simulink model "Simulatie"  (R2018b)
settings: Solver=FixedStepAuto  StartTime=0.0  StopTime=10  FixedStep=1e-5  RelTol=1e-3
values from neighbouring files (symbols this model uses):
  A = [-(bm*(n^2) + bg)/(Jm*(n^2) + Jg) Kt*n/(Jm*(n^2) + Jg) ... (first row only)    [DC_motor_geared_integral_discrete_sysid23.m]    (also in DC_motor_geared_lqr_discrete_sysid23.m; finalScript.m; finalScriptV2.m; precompensatorVSintegrator.m)
  Ad = sysdi.A    [DC_motor_geared_integral_discrete_sysid23.m]    (also in DC_motor_geared_lqr_discrete_sysid23.m = sysd.A; finalScript.m; finalScriptV2.m)
  B = [0 ... (first row only)    [DC_motor_geared_integral_discrete_sysid23.m]    (also in DC_motor_geared_lqr_discrete_sysid23.m; finalScript.m; finalScriptV2.m; precompensatorVSintegrator.m)
  Bd = sysdi.B    [DC_motor_geared_integral_discrete_sysid23.m]    (also in DC_motor_geared_lqr_discrete_sysid23.m = sysd.B; finalScript.m; finalScriptV2.m)
  C = [1 0]    [DC_motor_geared_integral_discrete_sysid23.m]    (also in DC_motor_geared_lqr_discrete_sysid23.m = eye(2); finalScript.m; finalScriptV2.m; precompensatorVSintegrator.m = eye(2))
  D = [0]    [DC_motor_geared_integral_discrete_sysid23.m]    (also in DC_motor_geared_lqr_discrete_sysid23.m = [0;0]; finalScript.m; finalScriptV2.m; precompensatorVSintegrator.m)
  Kc = lqr(sysd,Q,R)    [DC_motor_geared_lqr_discrete_sysid23.m]    (also in precompensatorVSintegrator.m = lqr(sysc,Q,R))
  n = 16.5    [DC_motor_geared_integral_discrete_sysid23.m]    (also in DC_motor_geared_lqr_discrete_sysid23.m; finalScript.m; finalScriptV2.m)
  Nbar = rscale(sys_ss,Kc)    [DC_motor_geared_lqr_discrete_sysid23.m]    (also in precompensatorVSintegrator.m; rscale.m = Nu + K*Nx)
  Tsc = 1/20000    (= 5e-05)    [DC_motor_geared_integral_discrete_sysid23.m]    (also in DC_motor_geared_lqr_discrete_sysid23.m = 1e-05; finalScript.m; finalScriptV2.m = 0.001)
undefined symbols (not defined in the file or in its folder): DiscIntNeverNeededParam, sigbuilder_block
libraries: powerlib_meascontrol x7, simulink x4, dspswit3 x4, dspsigops x1, peLuenbergerObserver x1, dspstat3 x1
settings Model: Creator=BooJC  LastModifiedBy=Roberto
settings DataIOCC: ExternalInput=v_motor_ts
settings DebuggingCC: LibraryContextMissingDiagnostic=none
settings SFSimCC: SimUseLocalCustomCode=off
settings RTWCC: RTWUseLocalCustomCode=off

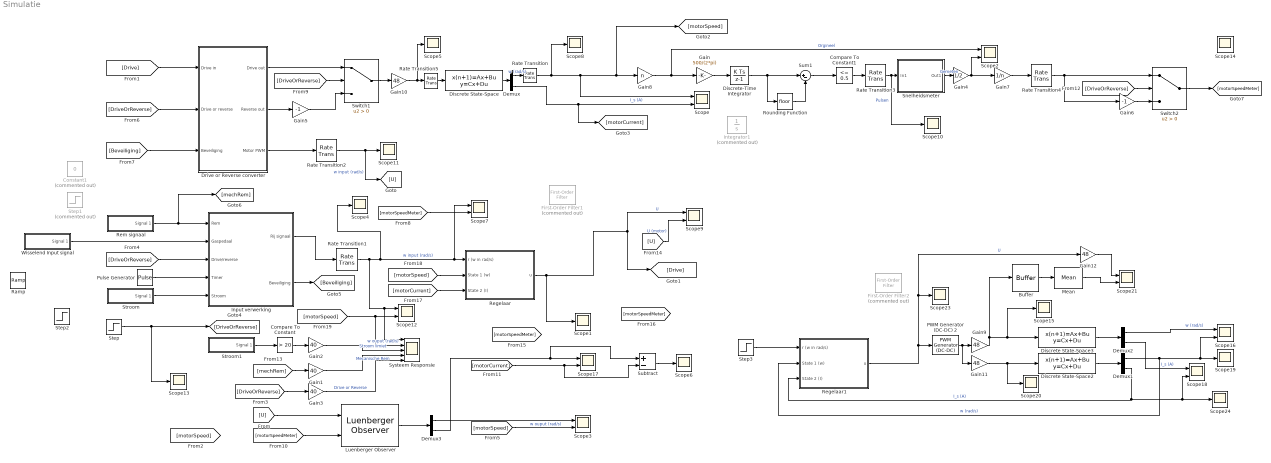
== system Simulatie ==
  Buffer : Buffer  N=1000  OutputFrames=off
  Compare To Constant : simulink/Logic and Bit Operations/Compare To Constant  relop=>  const=20  OutDataTypeStr=boolean
  Compare To Constant1 : simulink/Logic and Bit Operations/Compare To Constant  relop=<=  const=0.5  OutDataTypeStr=boolean
  Constant1 : Constant  Commented=on  Value=0
  Demux{,1..3} (4 alike) : Demux  Outputs=2
  Discrete State-Space : DiscreteStateSpace  A=Ad  B=Bd  C=eye(2)  D=[0; 0]  SampleTime=Tsc
  Discrete State-Space2 : DiscreteStateSpace  A=Ad  B=Bd  C=eye(2)  D=[0; 0]  SampleTime=1/(1e5)
  Discrete State-Space3 : DiscreteStateSpace  A=Ad  B=Bd  C=eye(2)  D=[0; 0]  SampleTime=1/(1e5)
  Discrete-Time Integrator : DiscreteIntegrator  SampleTime=-1  ICPrevOutput=DiscIntNeverNeededParam  ICPrevScaledInput=DiscIntNeverNeededParam
  Drive or Reverse converter : Subsystem
  First-Order Filter1 : powerlib_meascontrol/Filters/First-Order Filter  Commented=on  FilterType=Lowpass  Tc=10e-2  Ts=Tsc  Initialize=on  Vac_Init=[0, 0, 50]  Vdc_Init=0  PlotResponse=off  FreqRange="[0,  200,  1]"
      settings: SourceProductName=Simscape Power Systems
  First-Order Filter2 : powerlib_meascontrol/Filters/First-Order Filter  Commented=on  FilterType=Lowpass  Tc=10e-2  Ts=Tsc*100  Initialize=on  Vac_Init=[0, 0, 50]  Vdc_Init=0  PlotResponse=off  FreqRange="[0,  200,  1]"
      settings: SourceProductName=Simscape Power Systems
  Gain : Gain  Gain=500/(2*pi)
  Gain1 : Gain  Gain=40
  Gain{9..12} (4 alike) : Gain  Gain=48
  Gain2 : Gain  Gain=40
  Gain3 : Gain  Gain=40
  Gain4 : Gain  Gain=1/2
  Gain5 : Gain  Gain=-1
  Gain6 : Gain  Gain=-1
  Gain7 : Gain  Gain=1/n
  Gain8 : Gain  Gain=n
  Input verwerking : Subsystem
  Integrator1 : Integrator  Commented=on
  Luenberger Observer : peLuenbergerObserver/Luenberger Observer  StateSpaceType=Discrete-time  Ad=Ad  Bd=Bd  Cd=[1 0]  Dd=0  A=A  B=B  C=C  D=D  ObserverDesign=Observer gain  Ld=L  DesiredEigenvalues=eigenVal  x0=[0 0]  Tsd=0.1  Ts=Tsc
  Mean : dspstat3/Mean  run=off  InputProcessing=Columns as channels (frame based)  reset_popup=None  directionMode=Entire input  dimension=1  roiEnable=off  roiType=Rectangles  roiPortion=Entire ROI  roiOutput=Individual statistics for each ROI  roiFlag=off  roundingMode=Floor  overflowMode=off  outputDataTypeStr=Inherit: Same as accumulator  outputMin=[]  outputMax=[]  outputLastDataTypeStr=Inherit: Same as accumulator
  PWM Generator (DC-DC) 2 : powerlib_meascontrol/Pulse & Signal Generators/PWM Generator (DC-DC)  Fsw=20e3  Ts=1/(1e5)
      settings: SourceProductName=Simscape Electrical
  Pulse Generator : DiscretePulseGenerator  SampleTime=1/2000
  Ramp : simulink/Sources/Ramp  slope=0.33  start=0  InitialOutput=0
  Rate Transition : RateTransition  OutPortSampleTime=1/100000
  Rate Transition{1..2,4..5} (4 alike) : RateTransition  OutPortSampleTime=Tsc
  Rate Transition3 : RateTransition  OutPortSampleTime=1/100000
  Regelaar : Subsystem
  Regelaar1 : Subsystem
  Rem signaal : Subsystem  Tag=STV Subsys  LoadFcn=sigbuilder_block('load');  StartFcn=sigbuilder_block('start');  StopFcn=sigbuilder_block('stop');  ClipboardFcn=sigbuilder_block('clipboard');  mask(Sigbuilder block){tuvar=[0:10]}
      mask help: Simulink:masks:SigbuilderBlock_MD
      mask init:
      | if ~strcmp(get_param(bdroot(gcbh),'SimulationStatus'),'stopped') tuvar = sigbuilder_block('maskInit'); end
      settings: CopyFcn=sigbuilder_block('copy');  DeleteFcn=sigbuilder_block('delete');  ModelCloseFcn=sigbuilder_block('modelClose');  PreSaveFcn=sigbuilder_block('preSave');  PauseFcn=sigbuilder_block('pause');  ContinueFcn=sigbuilder_block('continue');  NameChangeFcn=sigbuilder_block('namechange');  OpenFcn=sigbuilder_block('open',[437.6 153 550.4 359.25 ]);  CloseFcn=sigbuilder_block('close');
      mask Display: plot(0, 0, 100, 100,[2, 2, 32, 32, 2], [68, 8, 8, 68, 68],[32, 2], [38, 38], [32, 19, 2],[53, 60, 44], [32, 17, 17, 2],[16, 16, 31, 31]);txt = getActiveGroup(gcbh);text(2, 100, txt,'verticalAlignment', 'top');
  Rounding Function : Rounding
  Scope{,2..3,7,9,12,16..18,21} (10 alike) : Scope  NumInputPorts=2
  Scope{1,4..6,8,10..11,13..15,19..20,23..24} (14 alike) : Scope
  Snelheidsmeter : Subsystem
  Step : Step  Time=50  Before=1  After=0  SampleTime=1/1000
  Step1 : Step  Commented=on  After=3.3  SampleTime=1/100000
  Step2 : Step  Time=0.1  After=0.5  SampleTime=0
  Step3 : Step  Time=0.1  After=30  SampleTime=1/1000
  Stroom : Subsystem  Tag=STV Subsys  LoadFcn=sigbuilder_block('load');  StartFcn=sigbuilder_block('start');  StopFcn=sigbuilder_block('stop');  ClipboardFcn=sigbuilder_block('clipboard');  mask(Sigbuilder block){tuvar=[0:10]}
      mask help: Simulink:masks:SigbuilderBlock_MD
      mask init:
      | if ~strcmp(get_param(bdroot(gcbh),'SimulationStatus'),'stopped') tuvar = sigbuilder_block('maskInit'); end
      settings: CopyFcn=sigbuilder_block('copy');  DeleteFcn=sigbuilder_block('delete');  ModelCloseFcn=sigbuilder_block('modelClose');  PreSaveFcn=sigbuilder_block('preSave');  PauseFcn=sigbuilder_block('pause');  ContinueFcn=sigbuilder_block('continue');  NameChangeFcn=sigbuilder_block('namechange');  OpenFcn=sigbuilder_block('open',[437.6 153 550.4 359.25 ]);  CloseFcn=sigbuilder_block('close');
      mask Display: plot(0, 0, 100, 100,[2, 2, 32, 32, 2], [68, 8, 8, 68, 68],[32, 2], [38, 38], [32, 19, 2],[53, 60, 44], [32, 17, 17, 2],[16, 16, 31, 31]);txt = getActiveGroup(gcbh);text(2, 100, txt,'verticalAlignment', 'top');
  Stroom1 : Subsystem  Tag=STV Subsys  LoadFcn=sigbuilder_block('load');  StartFcn=sigbuilder_block('start');  StopFcn=sigbuilder_block('stop');  ClipboardFcn=sigbuilder_block('clipboard');  mask(Sigbuilder block){tuvar=[0:10]}
      mask help: Simulink:masks:SigbuilderBlock_MD
      mask init:
      | if ~strcmp(get_param(bdroot(gcbh),'SimulationStatus'),'stopped') tuvar = sigbuilder_block('maskInit'); end
      settings: CopyFcn=sigbuilder_block('copy');  DeleteFcn=sigbuilder_block('delete');  ModelCloseFcn=sigbuilder_block('modelClose');  PreSaveFcn=sigbuilder_block('preSave');  PauseFcn=sigbuilder_block('pause');  ContinueFcn=sigbuilder_block('continue');  NameChangeFcn=sigbuilder_block('namechange');  OpenFcn=sigbuilder_block('open',[437.6 153 550.4 359.25 ]);  CloseFcn=sigbuilder_block('close');
      mask Display: plot(0, 0, 100, 100,[2, 2, 32, 32, 2], [68, 8, 8, 68, 68],[32, 2], [38, 38], [32, 19, 2],[53, 60, 44], [32, 17, 17, 2],[16, 16, 31, 31]);txt = getActiveGroup(gcbh);text(2, 100, txt,'verticalAlignment', 'top');
  Subtract : Sum  Inputs=+-
  Sum1 : Sum  Inputs=|+-
  Switch1 : Switch  Criteria=u2 > Threshold
  Switch2 : Switch  Criteria=u2 > Threshold
  Systeem Responsie : Scope  NumInputPorts=5
  Wisselend Input signal : Subsystem  Tag=STV Subsys  LoadFcn=sigbuilder_block('load');  StartFcn=sigbuilder_block('start');  StopFcn=sigbuilder_block('stop');  ClipboardFcn=sigbuilder_block('clipboard');  mask(Sigbuilder block){tuvar=[0:10]}
      mask help: Simulink:masks:SigbuilderBlock_MD
      mask init:
      | if ~strcmp(get_param(bdroot(gcbh),'SimulationStatus'),'stopped') tuvar = sigbuilder_block('maskInit'); end
      settings: CopyFcn=sigbuilder_block('copy');  DeleteFcn=sigbuilder_block('delete');  ModelCloseFcn=sigbuilder_block('modelClose');  PreSaveFcn=sigbuilder_block('preSave');  PauseFcn=sigbuilder_block('pause');  ContinueFcn=sigbuilder_block('continue');  NameChangeFcn=sigbuilder_block('namechange');  OpenFcn=sigbuilder_block('open',[437.6 153 550.4 359.25 ]);  CloseFcn=sigbuilder_block('close');
      mask Display: plot(0, 0, 100, 100,[2, 2, 32, 32, 2], [68, 8, 8, 68, 68],[32, 2], [38, 38], [32, 19, 2],[53, 60, 44], [32, 17, 17, 2],[16, 16, 31, 31]);txt = getActiveGroup(gcbh);text(2, 100, txt,'verticalAlignment', 'top');
  wires:
  Rate Transition1/1 -> Scope4/1, Scope7/1, Regelaar/1(r (w in rad/s)), Scope12/1, Systeem Responsie/1  "w input (rad/s)"
  Demux/1 -> Rate Transition/1  "w (rad/s)"
  Demux/2 -> [motorCurrent], Scope/2  "I_s (A)"
  Rem signaal/1(Signal 1) -> Input verwerking/1(Rem), [mechRem]
  [DriveOrReverse] -> Input verwerking/3(Drive/reverse)
  [Drive] -> Drive or Reverse converter/1(Drive in)
  [DriveOrReverse] -> Drive or Reverse converter/2(Drive or reverse)
  Step/1 -> Scope13/1, [DriveOrReverse]
  [motorSpeed] -> Scope12/2, Systeem Responsie/2  "w ouput (rad/s)"
  Luenberger Observer/1 -> Demux3/1
  Demux3/2 -> Subtract/1, Scope17/1
  [motorCurrent] -> Subtract/2, Scope17/2
  [motorSpeed] -> Scope3/2  "w ouput (rad/s)"
  Demux3/1 -> Scope3/1
  Compare To Constant/1 -> Gain2/1
  [mechRem] -> Gain1/1
  Gain2/1 -> Systeem Responsie/3  "Stroom limiet"
  Gain1/1 -> Systeem Responsie/4  "Mecanische Rem"
  Rate Transition2/1 -> [U], Scope11/1  "w input (rad/s)"
  Wisselend Input signal/1(Signal 1) -> Input verwerking/2(Gaspedaal)
  [motorSpeedMeter] -> Scope7/2
  Compare To Constant1/1 -> Rate Transition3/1
  Discrete-Time Integrator/1 -> Rounding Function/1, Sum1/1
  Rounding Function/1 -> Sum1/2
  Sum1/1 -> Compare To Constant1/1
  Rate Transition3/1 -> Scope10/1, Snelheidsmeter/1(In1)  "Pulsen"
  [motorSpeedMeter] -> Luenberger Observer/2
  Snelheidsmeter/1(Out1) -> Gain4/1  "Gemeten"
  Discrete State-Space/1 -> Demux/1
  Gain8/1 -> Scope2/1, Gain/1  "Orgineel"
  Gain7/1 -> Rate Transition4/1
  Input verwerking/1(Rij signaal) -> Rate Transition1/1
  Gain10/1 -> Scope5/1, Rate Transition5/1
  Gain/1 -> Discrete-Time Integrator/1
  [U] -> Luenberger Observer/1
  Subtract/1 -> Scope6/1
  Rate Transition/1 -> Scope/1, [motorSpeed], Gain8/1, Scope8/1
  Regelaar/1(u) -> [Drive], Scope9/1, Scope1/1  "U"
  Rate Transition5/1 -> Discrete State-Space/1
  [U] -> Scope9/2  "U (motor)"
  [DriveOrReverse] -> Gain3/1
  Gain3/1 -> Systeem Responsie/5  "Drive or Reverse"
  Gain4/1 -> Gain7/1, Scope2/2
  Stroom/1(Signal 1) -> Input verwerking/5(Stroom)
  Pulse Generator/1 -> Input verwerking/4(Timer)
  Input verwerking/2(Beveiliging) -> [Beveiliging]
  [Beveiliging] -> Drive or Reverse converter/3(Beveiliging)
  Stroom1/1(Signal 1) -> Compare To Constant/1
  Drive or Reverse converter/3(Motor PWM) -> Rate Transition2/1
  Drive or Reverse converter/1(Drive out) -> Switch1/1
  Drive or Reverse converter/2(Reverse out) -> Gain5/1
  Switch1/1 -> Gain10/1
  [DriveOrReverse] -> Switch1/2
  Gain5/1 -> Switch1/3
  Gain6/1 -> Switch2/3
  Rate Transition4/1 -> Gain6/1, Switch2/1
  [DriveOrReverse] -> Switch2/2
  Switch2/1 -> [motorSpeedMeter]
  [motorSpeed] -> Regelaar/2(State 1 (w))
  [motorCurrent] -> Regelaar/3(State 2 (I))
  Gain11/1 -> Discrete State-Space2/1, Scope20/1
  Discrete State-Space2/1 -> Demux1/1
  Demux1/2 -> Scope18/2, Scope24/1, Regelaar1/3(State 2 (I))  "I_s (A)"
  Demux1/1 -> Scope16/2, Scope19/1, Regelaar1/2(State 1 (w))  "w (rad/s)"
  Step3/1 -> Regelaar1/1(r (w in rad/s))
  Mean/1 -> Scope21/2
  Regelaar1/1(u) -> PWM Generator (DC-DC) 2/1, Gain12/1, Scope23/1  "U"
  Buffer/1 -> Mean/1
  PWM Generator (DC-DC) 2/1 -> Gain11/1, Gain9/1
  Discrete State-Space3/1 -> Demux2/1
  Demux2/1 -> Scope16/1  "w (rad/s)"
  Demux2/2 -> Scope18/1  "I_s (A)"
  Gain9/1 -> Scope15/1, Discrete State-Space3/1, Buffer/1
  Gain12/1 -> Scope21/1

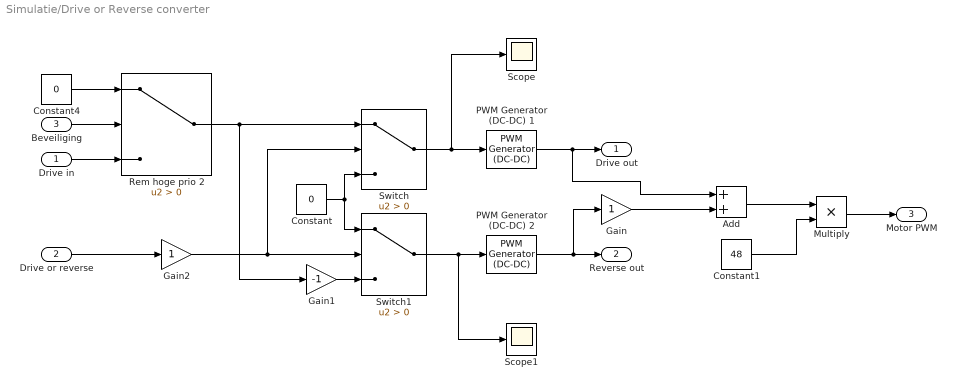
== system Simulatie/Drive or Reverse converter ==
  Drive in : Inport
  Drive or reverse : Inport  Port=2
  Beveiliging : Inport  Port=3
  Add : Sum
  Constant : Constant  Value=0
  Constant1 : Constant  Value=48
  Constant4 : Constant  Value=0
  Gain : Gain
  Gain1 : Gain  Gain=-1
  Gain2 : Gain
  Multiply : Product
  PWM Generator (DC-DC) 1 : powerlib_meascontrol/Pulse & Signal Generators/PWM Generator (DC-DC)  Fsw=20e3  Ts=1/(1e5)
      settings: SourceProductName=Simscape Electrical
  PWM Generator (DC-DC) 2 : powerlib_meascontrol/Pulse & Signal Generators/PWM Generator (DC-DC)  Fsw=20e3  Ts=1/(1e5)
      settings: SourceProductName=Simscape Electrical
  Rem hoge prio 2 : Switch  Criteria=u2 > Threshold
  Scope : Scope
  Scope1 : Scope
  Switch : Switch  Criteria=u2 > Threshold
  Switch1 : Switch  Criteria=u2 > Threshold
  Drive out : Outport
  Reverse out : Outport  Port=2
  Motor PWM : Outport  Port=3
  wires:
  Gain1/1 -> Switch1/3
  Switch1/1 -> Scope1/1, PWM Generator (DC-DC) 2/1
  Switch/1 -> Scope/1, PWM Generator (DC-DC) 1/1
  Constant4/1 -> Rem hoge prio 2/1
  Constant/1 -> Switch1/1, Switch/3
  Rem hoge prio 2/1 -> Gain1/1, Switch/1
  Drive in/1 -> Rem hoge prio 2/3
  Beveiliging/1 -> Rem hoge prio 2/2
  PWM Generator (DC-DC) 1/1 -> Add/1, Drive out/1
  PWM Generator (DC-DC) 2/1 -> Reverse out/1, Gain/1
  Gain/1 -> Add/2
  Constant1/1 -> Multiply/2
  Add/1 -> Multiply/1
  Gain2/1 -> Switch/2, Switch1/2
  Drive or reverse/1 -> Gain2/1
  Multiply/1 -> Motor PWM/1

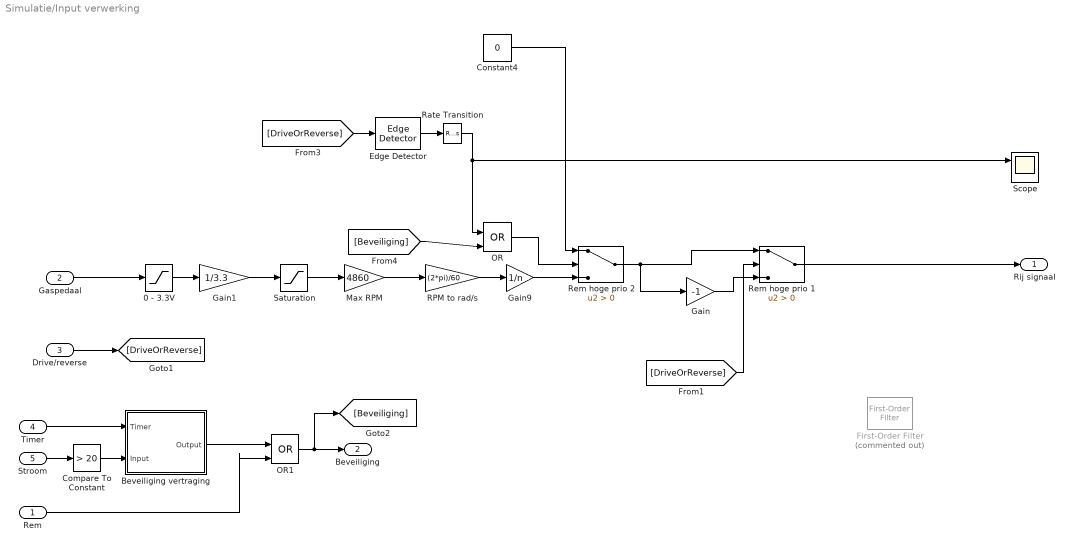
== system Simulatie/Input verwerking ==
  Rem : Inport
  Gaspedaal : Inport  Port=2
  Drive/reverse : Inport  Port=3
  Timer : Inport  Port=4
  Stroom : Inport  Port=5
  0 - 3.3V : Saturate  UpperLimit=3.3  LowerLimit=0
  Beveiliging vertraging : Subsystem
  Compare To Constant : simulink/Logic and Bit Operations/Compare To Constant  relop=>  const=20  OutDataTypeStr=boolean
  Constant4 : Constant  Value=0
  Edge Detector : powerlib_meascontrol/Logic/Edge Detector  model=Either  ic=0  Ts=1/1000
      settings: SourceProductName=Simscape Power Systems  SourceProductBaseCode=PS
  First-Order Filter : powerlib_meascontrol/Filters/First-Order Filter  Commented=on  FilterType=Lowpass  Tc=10e-2  Ts=0  Initialize=on  Vac_Init=[0, 0, 60]  Vdc_Init=0  PlotResponse=off  FreqRange="[0,  200,  1]"
      settings: SourceProductName=Simscape Power Systems
  Gain : Gain  Gain=-1
  Gain1 : Gain  Gain=1/3.3
  Gain9 : Gain  Gain=1/n
  Max RPM : Gain  Gain=4860
  OR : Logic  Operator=OR  IconShape=distinctive  AllPortsSameDT=off  OutDataTypeStr=boolean
  OR1 : Logic  Operator=OR  IconShape=distinctive  AllPortsSameDT=off  OutDataTypeStr=boolean
  RPM to rad/s : Gain  Gain=(2*pi)/60
  Rate Transition : RateTransition  OutPortSampleTime=0.2
  Rem hoge prio 1 : Switch  Criteria=u2 > Threshold
  Rem hoge prio 2 : Switch  Criteria=u2 > Threshold
  Saturation : Saturate  UpperLimit=inf  LowerLimit=0
  Scope : Scope  NumInputPorts=2
  Rij signaal : Outport
  Beveiliging : Outport  Port=2
  wires:
  Constant4/1 -> Rem hoge prio 2/1
  0 - 3.3V/1 -> Gain1/1
  Max RPM/1 -> RPM to rad/s/1
  Saturation/1 -> Max RPM/1
  RPM to rad/s/1 -> Gain9/1
  Gaspedaal/1 -> 0 - 3.3V/1
  Drive/reverse/1 -> [DriveOrReverse]
  Gain1/1 -> Saturation/1
  OR/1 -> Rem hoge prio 2/2
  [DriveOrReverse] -> Edge Detector/1
  Edge Detector/1 -> Rate Transition/1
  Rate Transition/1 -> OR/1, Scope/1
  Timer/1 -> Beveiliging vertraging/1(Timer)
  Stroom/1 -> Compare To Constant/1
  Beveiliging vertraging/1(Output) -> OR1/1
  Rem/1 -> OR1/2
  OR1/1 -> [Beveiliging], Beveiliging/1
  [Beveiliging] -> OR/2
  Compare To Constant/1 -> Beveiliging vertraging/2(Input)
  Gain9/1 -> Rem hoge prio 2/3
  Rem hoge prio 1/1 -> Rij signaal/1
  Rem hoge prio 2/1 -> Gain/1, Rem hoge prio 1/1
  Gain/1 -> Rem hoge prio 1/3
  [DriveOrReverse] -> Rem hoge prio 1/2

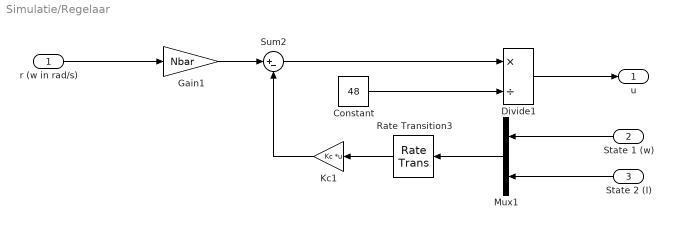
== system Simulatie/Regelaar ==
  r (w in rad/s) : Inport
  State 1 (w) : Inport  Port=2
  State 2 (I) : Inport  Port=3
  Constant : Constant  Value=48
  Divide1 : Product  Inputs=*/
  Gain1 : Gain  Gain=Nbar
  Kc1 : Gain  Gain=Kc  Multiplication=Matrix(K*u)
  Mux1 : Mux  Inputs=2
  Rate Transition3 : RateTransition  OutPortSampleTime=Tsc
  Sum2 : Sum  Inputs=|+-
  u : Outport
  wires:
  Mux1/1 -> Rate Transition3/1
  Sum2/1 -> Divide1/1
  Rate Transition3/1 -> Kc1/1
  State 1 (w)/1 -> Mux1/1
  Kc1/1 -> Sum2/2
  Constant/1 -> Divide1/2
  Gain1/1 -> Sum2/1
  Divide1/1 -> u/1
  r (w in rad/s)/1 -> Gain1/1
  State 2 (I)/1 -> Mux1/2

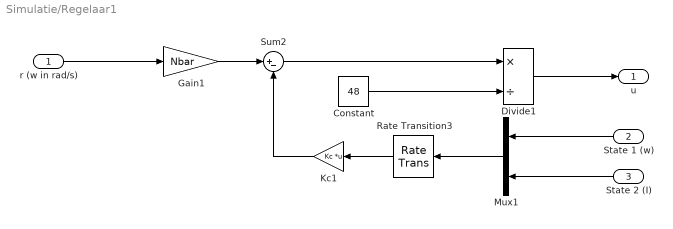
== system Simulatie/Regelaar1 ==
  r (w in rad/s) : Inport
  State 1 (w) : Inport  Port=2
  State 2 (I) : Inport  Port=3
  Constant : Constant  Value=48
  Divide1 : Product  Inputs=*/
  Gain1 : Gain  Gain=Nbar
  Kc1 : Gain  Gain=Kc  Multiplication=Matrix(K*u)
  Mux1 : Mux  Inputs=2
  Rate Transition3 : RateTransition  OutPortSampleTime=Tsc
  Sum2 : Sum  Inputs=|+-
  u : Outport
  wires:
  Mux1/1 -> Rate Transition3/1
  Sum2/1 -> Divide1/1
  Rate Transition3/1 -> Kc1/1
  State 1 (w)/1 -> Mux1/1
  Kc1/1 -> Sum2/2
  Constant/1 -> Divide1/2
  Gain1/1 -> Sum2/1
  Divide1/1 -> u/1
  r (w in rad/s)/1 -> Gain1/1
  State 2 (I)/1 -> Mux1/2

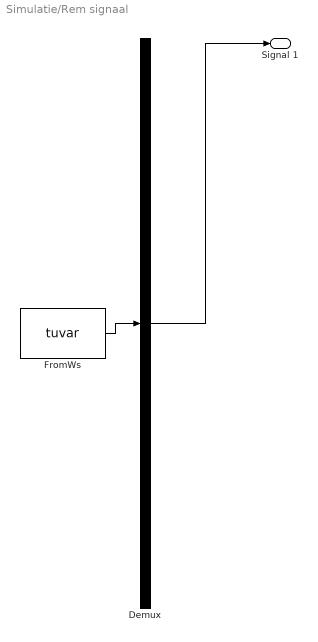
== system Simulatie/Rem signaal ==
  Demux : Demux  Tag=STV Demux  Outputs=1
  FromWs : FromWorkspace  Tag=STV FromWs  VariableName=tuvar  SampleTime=0
      SigBuilderData=|
      | common.afterFinalStr = 'Extrapolate'
      | common.sampleTime = 0
      | dataSet.timeRange = [0 10]
      | dataSet.name = 'Group 1'
      | sbobj.Groups.Name = 'Group 1'
      | sbobj.Groups.Signals.Name = 'Signal 1'
      | sbobj.Groups.Signals.XData = [0 6 6 7 7 10]
      | sbobj.Groups.Signals.YData = [0 0 1 1 0 0]
  Signal 1 : Outport  Tag=STV Outport
  wires:
  Demux/1 -> Signal 1/1
  FromWs/1 -> Demux/1

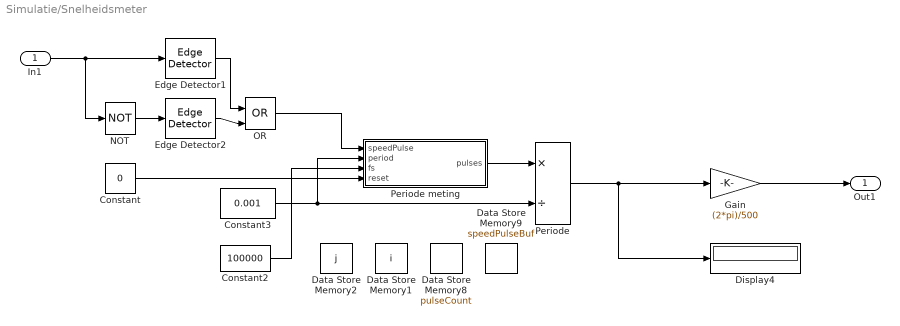
== system Simulatie/Snelheidsmeter ==
  In1 : Inport
  Constant : Constant  Value=0
  Constant2 : Constant  Value=100000
  Constant3 : Constant  Value=0.001
  Data Store Memory1 : DataStoreMemory  DataStoreName=i  ReadBeforeWriteMsg=warning  WriteAfterWriteMsg=warning  WriteAfterReadMsg=warning  InitialValue=1  ShowAdditionalParam=off  OutDataTypeStr=uint32
  Data Store Memory2 : DataStoreMemory  DataStoreName=j  ReadBeforeWriteMsg=warning  WriteAfterWriteMsg=warning  WriteAfterReadMsg=warning  InitialValue=2  ShowAdditionalParam=off  OutDataTypeStr=uint32
  Data Store Memory8 : DataStoreMemory  DataStoreName=pulseCount  ReadBeforeWriteMsg=warning  WriteAfterWriteMsg=warning  WriteAfterReadMsg=warning  ShowAdditionalParam=off  OutDataTypeStr=uint32
  Data Store Memory9 : DataStoreMemory  DataStoreName=speedPulseBuf  ReadBeforeWriteMsg=warning  WriteAfterWriteMsg=warning  WriteAfterReadMsg=warning  ShowAdditionalParam=off  OutDataTypeStr=uint8  Dimensions=10001
  Display4 : Display
  Edge Detector1 : dspswit3/Edge Detector  InputProcessing=Columns as channels (frame based)
      settings: SourceProductName=DSP System Toolbox  SourceProductBaseCode=DS
  Edge Detector2 : dspswit3/Edge Detector  InputProcessing=Columns as channels (frame based)
      settings: SourceProductName=DSP System Toolbox  SourceProductBaseCode=DS
  Gain : Gain  Gain=(2*pi)/500
  NOT : Logic  Operator=NOT  IconShape=distinctive  AllPortsSameDT=off  OutDataTypeStr=boolean
  OR : Logic  Operator=OR  IconShape=distinctive  AllPortsSameDT=off  OutDataTypeStr=boolean
  Periode : Product  Inputs=*/
  Periode meting : MATLAB Function  TreatAsAtomicUnit=on
  Out1 : Outport
  wires:
  Constant3/1 -> Periode/2, Periode meting/2(period)
  Periode/1 -> Gain/1, Display4/1
  Constant2/1 -> Periode meting/3(fs)
  Periode meting/1(pulses) -> Periode/1
  In1/1 -> NOT/1, Edge Detector1/1
  Gain/1 -> Out1/1
  Constant/1 -> Periode meting/4(reset)
  OR/1 -> Periode meting/1(speedPulse)
  Edge Detector1/1 -> OR/1
  Edge Detector2/1 -> OR/2
  NOT/1 -> Edge Detector2/1

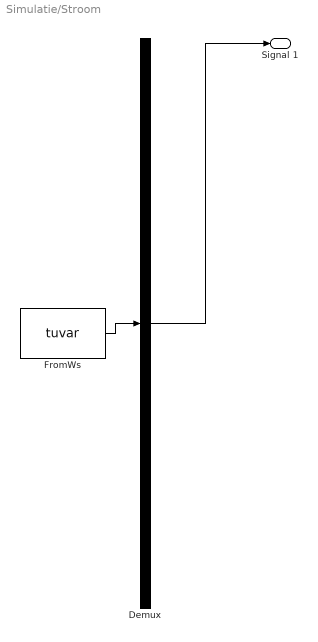
== system Simulatie/Stroom ==
  Demux : Demux  Tag=STV Demux  Outputs=1
  FromWs : FromWorkspace  Tag=STV FromWs  VariableName=tuvar  SampleTime=0
      SigBuilderData=|
      | common.afterFinalStr = 'Extrapolate'
      | common.sampleTime = 0
      | dataSet.timeRange = [0 10]
      | dataSet.name = 'Group 1'
      | sbobj.Groups.Name = 'Group 1'
      | sbobj.Groups.Signals.Name = 'Signal 1'
      | sbobj.Groups.Signals.XData = [0 1 1.5 2 7 10]
      | sbobj.Groups.Signals.YData = [0 0 30 0 0 0]
  Signal 1 : Outport  Tag=STV Outport
  wires:
  Demux/1 -> Signal 1/1
  FromWs/1 -> Demux/1

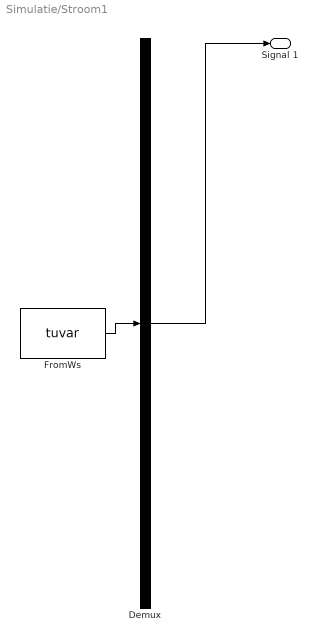
== system Simulatie/Stroom1 ==
  Demux : Demux  Tag=STV Demux  Outputs=1
  FromWs : FromWorkspace  Tag=STV FromWs  VariableName=tuvar  SampleTime=0
      SigBuilderData=|
      | common.afterFinalStr = 'Extrapolate'
      | common.sampleTime = 0
      | dataSet.timeRange = [0 10]
      | dataSet.name = 'Group 1'
      | sbobj.Groups.Name = 'Group 1'
      | sbobj.Groups.Signals.Name = 'Signal 1'
      | sbobj.Groups.Signals.XData = [0 1 1.5 2 7 10]
      | sbobj.Groups.Signals.YData = [0 0 30 0 0 0]
  Signal 1 : Outport  Tag=STV Outport
  wires:
  Demux/1 -> Signal 1/1
  FromWs/1 -> Demux/1

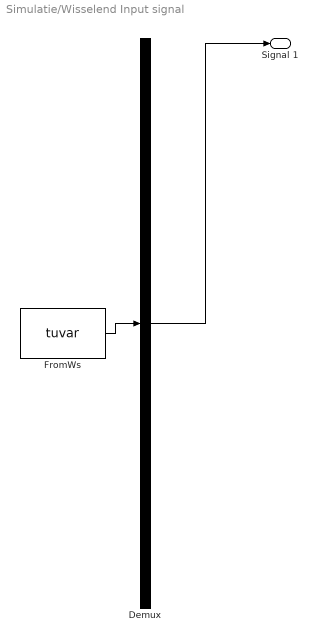
== system Simulatie/Wisselend Input signal ==
  Demux : Demux  Tag=STV Demux  Outputs=1
  FromWs : FromWorkspace  Tag=STV FromWs  VariableName=tuvar  SampleTime=0
      SigBuilderData=|
      | common.afterFinalStr = 'Extrapolate'
      | common.sampleTime = 0
      | dataSet.timeRange = [0 10]
      | dataSet.name = 'Group 1'
      | sbobj.Groups.Name = 'Group 1'
      | sbobj.Groups.Signals.Name = 'Signal 1'
      | sbobj.Groups.Signals.XData = [0 0.56 1 1 2 2 3 3 4 4 10]
      | sbobj.Groups.Signals.YData = [0 4 0 3.3 3.3 1 0 3.3 3.3 0 5]
  Signal 1 : Outport  Tag=STV Outport
  wires:
  Demux/1 -> Signal 1/1
  FromWs/1 -> Demux/1

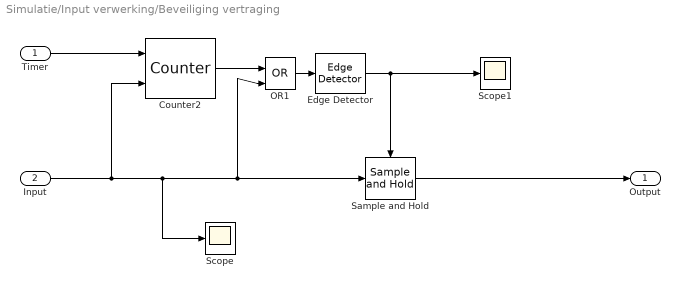
== system Simulatie/Input verwerking/Beveiliging vertraging ==
  Timer : Inport
  Input : Inport  Port=2
  Counter2 : dspswit3/Counter  Direction=Up  CountEvent=Rising edge  CounterSize=User defined  MaxCount=300  InitialCount=0  Output=Hit  HitValue=300  ResetInput=on  SamplesPerFrame=1  Ts=1  CntDtype=double  HitDtype=Logical
  Edge Detector : dspswit3/Edge Detector  InputProcessing=Columns as channels (frame based)
      settings: SourceProductName=DSP System Toolbox  SourceProductBaseCode=DS
  OR1 : Logic  Operator=OR  IconShape=distinctive  AllPortsSameDT=off  OutDataTypeStr=boolean
  Sample and Hold : dspsigops/Sample and Hold  trig=Rising edge  initCond=0  latchinput=off
  Scope : Scope
  Scope1 : Scope
  Output : Outport
  wires:
  Timer/1 -> Counter2/1
  Sample and Hold/1 -> Output/1
  OR1/1 -> Edge Detector/1
  Input/1 -> Counter2/2, Scope/1, OR1/2, Sample and Hold/1
  Edge Detector/1 -> Scope1/1, Sample and Hold/Trigger
  Counter2/1 -> OR1/1

== matlab function Simulatie/Snelheidsmeter/Periode meting ==
  data: speedPulse input; pulses output; speedPulseBuf data_store_memory; pulseCount data_store_memory; period input; i data_store_memory; fs input; j data_store_memory; reset input
function pulses = fcn(speedPulse,period, fs, reset)

global pulseCount;
global speedPulseBuf;
global i;
global j;

if reset == 1
    speedPulseBuf = uint8(zeros(size(speedPulseBuf)));
end

bufTime = period*fs + 1;

if i > bufTime
    i = uint32(1);
end

if j > bufTime
    j = uint32(1);
end

speedPulseBuf(i) = speedPulse;
pulseCount = pulseCount + uint32(speedPulse);
pulseCount = pulseCount - uint32(speedPulseBuf(j));

i = i + 1;
j = j + 1;

pulses = pulseCount;
